simulink model "forcetosbcomm_two"  (R2014a)
settings: Solver=ode1  StartTime=0.0  StopTime=inf  FixedStep=0.001  RelTol=1e-3
undefined symbols (not defined in the file): localhost, simget
libraries: rtai_utilities x2, jr3lib x2, rtai_devices x2, sfbc_lib x1
settings Model: Creator=wirnshofer  LastModifiedBy=wirnshofer
settings DataIOCC: SignalLoggingSaveFormat=ModelDataLogs
settings RTWCC: SystemTargetFile=prt.tlc  TemplateMakefile=prt.tmf  Description=Linux PREEMPT_RT Real-Time Target  ProcessScript=prt_make_rtw_hook
settings STFCustomTargetCC: TargetLangStandard=C99 (ISO)  CodeReplacementLibrary=GNU C99 extensions  ModelReferenceCompliant=off  ConcurrentExecutionCompliant=off  MatFileLogging=on  SystemTargetFile=prt.tlc
settings GRTTargetCC: TargetLangStandard=C99 (ISO)  CodeReplacementLibrary=GNU C99 extensions  ModelReferenceCompliant=off  ParMdlRefBuildCompliant=off  CompOptLevelCompliant=off  ConcurrentExecutionCompliant=off  CombineOutputUpdateFcns=off  CPPClassGenCompliant=off  GRTInterface=on

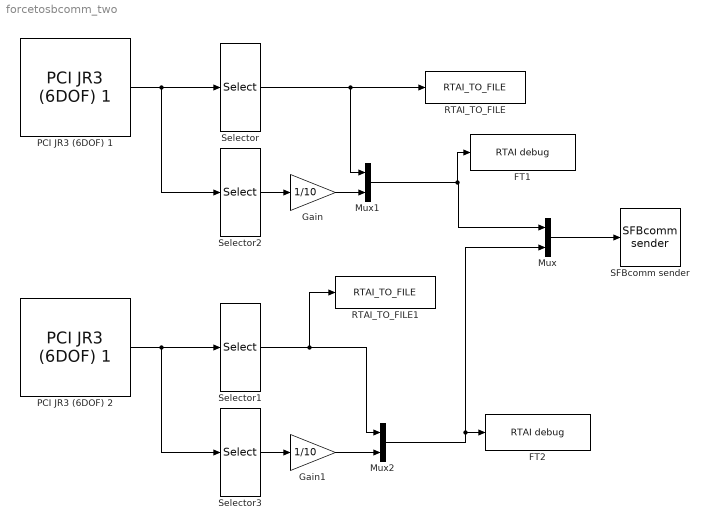
== system forcetosbcomm_two ==
  FT1 : rtai_utilities/RTAI debug  rate=1
  FT2 : rtai_utilities/RTAI debug  rate=1
  Gain : Gain  Gain=1/10
  Gain1 : Gain  Gain=1/10
  Mux : Mux  Inputs=2
  Mux1 : Mux  Inputs=2
  Mux2 : Mux  Inputs=2
  PCI JR3 (6DOF) 1 : jr3lib/PCI JR3 (6DOF) 1  bd_number=0  filter_nr=1  sampletime=simget(bdroot,'FixedStep')  begin_reset=on
  PCI JR3 (6DOF) 2 : jr3lib/PCI JR3 (6DOF) 1  bd_number=1  filter_nr=1  sampletime=simget(bdroot,'FixedStep')  begin_reset=on
  RTAI_TO_FILE : rtai_devices/RTAI_TO_FILE  N=3  InType=double  FileName='F1.dat'  FpOutStr='%f '  TStartStop=[1.1 50]  T=0.001  Confirm=off  Cutoff=off
  RTAI_TO_FILE1 : rtai_devices/RTAI_TO_FILE  N=3  InType=double  FileName='F2.dat'  FpOutStr='%f '  TStartStop=[1.1 50]  T=0.001  Confirm=off  Cutoff=off
  SFBcomm sender : sfbc_lib/SFBcomm sender  localPort=11112  streamID=1  remoteSettings=localhost:14531  portNames=A  connectTimeout=200  sampleTime=-1
  Selector : Selector  InputPortWidth=6  Indices=[1 2 3]
  Selector1 : Selector  InputPortWidth=6  Indices=[1 2 3]
  Selector2 : Selector  InputPortWidth=6  Indices=4:6
  Selector3 : Selector  InputPortWidth=6  Indices=4:6
  wires:
  PCI JR3 (6DOF) 1/1 -> Selector2/1, Selector/1
  Mux/1 -> SFBcomm sender/1
  Selector/1 -> Mux1/1, RTAI_TO_FILE/1
  Selector2/1 -> Gain/1
  Gain/1 -> Mux1/2
  PCI JR3 (6DOF) 2/1 -> Selector3/1, Selector1/1
  Selector1/1 -> RTAI_TO_FILE1/1, Mux2/1
  Selector3/1 -> Gain1/1
  Gain1/1 -> Mux2/2
  Mux1/1 -> FT1/1, Mux/1
  Mux2/1 -> Mux/2, FT2/1
